simulink model "table_test_2019b"  (R2019b)
settings: Solver=FixedStepAuto  StartTime=0.0  StopTime=200  RelTol=1e-3
InitFcn:
  | simin.time = [];
  | simin.signals.values = [10:5:90]';
libraries: mbedblockslib x5, simulink x1
settings Model: SimulationMode=external  SILPILModeSetting=veronly  ExtModeTrigDuration=10  Creator=The MathWorks, Inc.  LastModifiedBy=User
settings SolverCC: PositivePriorityOrder=on
settings DataIOCC: ReturnWorkspaceOutputs=off
settings OptimizationCC: MaxStackSize=64
settings DebuggingCC: ParameterTunabilityLossMsg=error  ArithmeticOperatorsInVariantConditions=warning
settings HardwareCC: ProdBitPerPointer=32  ProdBitPerSizeT=32  ProdBitPerPtrDiffT=32  ProdLargestAtomicInteger=Long  ProdLargestAtomicFloat=Double  ProdWordSize=32  ProdHWDeviceType=ARM Compatible->ARM Cortex  UseEmbeddedCoderFeatures=off
settings ModelReferenceCC: ModelReferenceNumInstancesAllowed=Single
settings SFSimCC: SimUseLocalCustomCode=off  CustomCodeUndefinedFunction=UseInterfaceOnly
settings RTWCC: SystemTargetFile=ert.tlc  HardwareBoard=STM32 Nucleo F767ZI  TemplateMakefile=ert_default_tmf  GenerateReport=on  RTWUseLocalCustomCode=off  Toolchain=GNU Tools for ARM Embedded Processors  LaunchReport=on
settings CodeAppCC: ForceParamTrailComments=on  OperatorAnnotations=on  StateflowObjectComments=on  MATLABSourceComments=on
settings ERTTargetCC: CodeReplacementLibrary=ARM Cortex-M (Optimized)  MultiwordLength=2048  ERTCustomFileBanners=off  SupportContinuousTime=on  SupportNonInlinedSFcns=on  RemoveResetFunc=off  ModelStepFunctionPrototypeControlCompliant=off  ExtMode=on  ExtModeTransport=3  ExtModeStaticAlloc=on  ExtModeStaticAllocSize=2000  ExtModeMexFile=ext_xcp  ExtModeMexArgs=1 4 460800  ExtModeIntrfLevel=Level2 - Open  ERTSrcFileBannerTemplate=codertarget_code_template.cgt  ERTHdrFileBannerTemplate=codertarget_code_template.cgt  ERTDataSrcFileTemplate=codertarget_code_template.cgt  ERTDataHdrFileTemplate=codertarget_code_template.cgt
settings ConfigComp: CovMetricSettings=dsw  CovHtmlReporting=on  CovSaveCumulativeToWorkspaceVar=on  CovSaveSingleToWorkspaceVar=on  CovShowResultsExplorer=off  CovExternalEMLEnable=off

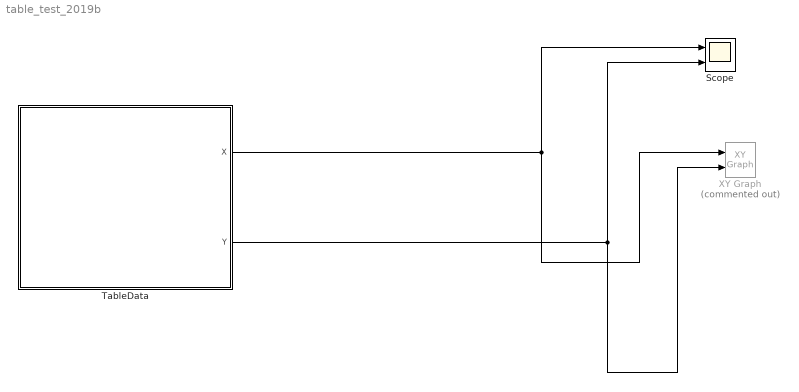
== system table_test_2019b ==
  Scope : Scope  NumInputPorts=2
  TableData : Subsystem
  XY Graph : simulink/Sinks/XY Graph  Commented=on  xmin=-1  xmax=1  ymin=-1  ymax=1  st=-1
  wires:
  TableData/1(X) -> Scope/1, XY Graph/1
  TableData/2(Y) -> Scope/2, XY Graph/2

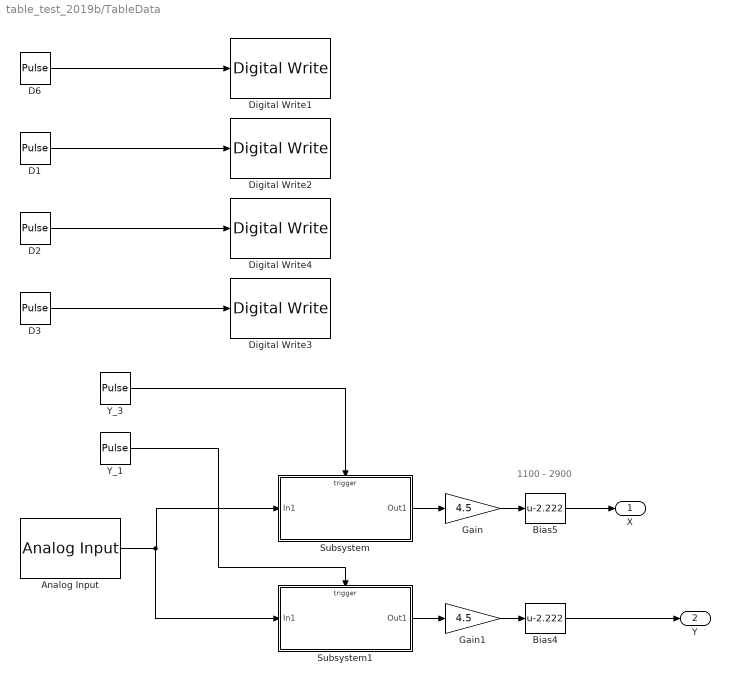
== system table_test_2019b/TableData ==
  note: 1100 - 2900
  Analog Input : mbedblockslib/Analog Input  Pin=PC_3  ReadResultsOnly=off  ConversionTriggerSource=Software  ExternalTriggerType=uint32( 0 )  OutputDataType=double  EnableConversionCompleteNotify=off  EnableOuputStatus=off  SampleTime=50e-6
      settings: SourceProductName=Simulink Coder Support Package for BBC microbit Board  SourceProductBaseCode=MICROBIT
  Bias4 : Bias  Bias=-2.222
  Bias5 : Bias  Bias=-2.222
  D1 : DiscretePulseGenerator  PulseType=Time based  Period=1000*10^(-6)  PulseWidth=50
  D2 : DiscretePulseGenerator  PulseType=Time based  Period=1000*10^(-6)  PulseWidth=50  PhaseDelay=500*10^(-6)
  D3 : DiscretePulseGenerator  PulseType=Time based  Period=1000*10^(-6)  PulseWidth=50  PhaseDelay=-250*10^(-6)
  D6 : DiscretePulseGenerator  PulseType=Time based  Period=1000*10^(-6)  PulseWidth=50  PhaseDelay=250*10^(-6)
  Digital Write1 : mbedblockslib/Digital Write  Pin=PD_6  Direction=output
      settings: SourceProductName=Simulink Coder Support Package for BBC microbit Board  SourceProductBaseCode=MICROBIT
  Digital Write2 : mbedblockslib/Digital Write  Pin=PD_5  Direction=output
      settings: SourceProductName=Simulink Coder Support Package for BBC microbit Board  SourceProductBaseCode=MICROBIT
  Digital Write3 : mbedblockslib/Digital Write  Pin=PD_3  Direction=output
      settings: SourceProductName=Simulink Coder Support Package for BBC microbit Board  SourceProductBaseCode=MICROBIT
  Digital Write4 : mbedblockslib/Digital Write  Pin=PD_4  Direction=output
      settings: SourceProductName=Simulink Coder Support Package for BBC microbit Board  SourceProductBaseCode=MICROBIT
  Gain : Gain  Gain=4.5
  Gain1 : Gain  Gain=4.5
  Subsystem : Subsystem
  Subsystem1 : Subsystem
  Y_1 : DiscretePulseGenerator  PulseType=Time based  Period=1000*10^(-6)  PhaseDelay=450*10^(-6)
  Y_3 : DiscretePulseGenerator  PulseType=Time based  Period=1000*10^(-6)  PhaseDelay=200*10^(-6)
  X : Outport
  Y : Outport  Port=2
  wires:
  Subsystem1/1(Out1) -> Gain1/1
  Bias4/1 -> Y/1
  D2/1 -> Digital Write4/1
  Analog Input/1 -> Subsystem1/1(In1), Subsystem/1(In1)
  D3/1 -> Digital Write3/1
  Y_1/1 -> Subsystem1/Trigger
  Subsystem/1(Out1) -> Gain/1
  D1/1 -> Digital Write2/1
  D6/1 -> Digital Write1/1
  Gain/1 -> Bias5/1
  Y_3/1 -> Subsystem/Trigger
  Gain1/1 -> Bias4/1
  Bias5/1 -> X/1

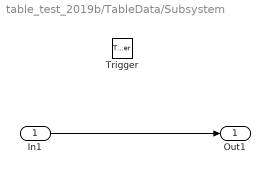
== system table_test_2019b/TableData/Subsystem ==
  In1 : Inport
  Trigger : TriggerPort  VariantControl=Variant  PortDimensions=1
  Out1 : Outport
  wires:
  In1/1 -> Out1/1

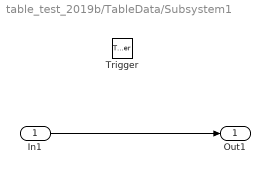
== system table_test_2019b/TableData/Subsystem1 ==
  In1 : Inport
  Trigger : TriggerPort  VariantControl=Variant  PortDimensions=1
  Out1 : Outport
  wires:
  In1/1 -> Out1/1
